simulink model "projet_RST_lineaire"  (R2023a)
settings: Solver=VariableStepAuto  StartTime=0.0  StopTime=1  RelTol=1e-3
undefined symbols (not defined in the file): R, S, T, Te
libraries: cstblocks x2
settings Model: Creator=leolebuhotel  LastModifiedBy=leolebuhotel

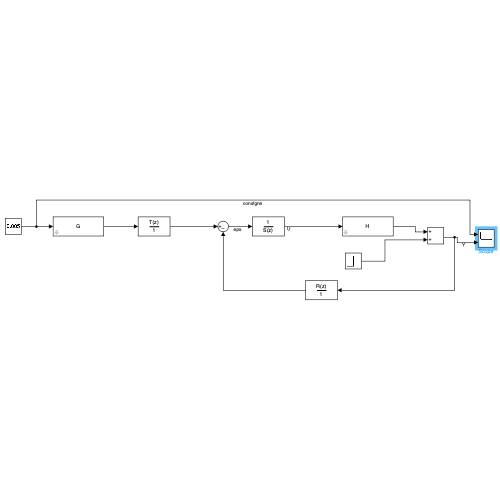
[thumbnail: Simulink's stored preview of the top-level diagram]
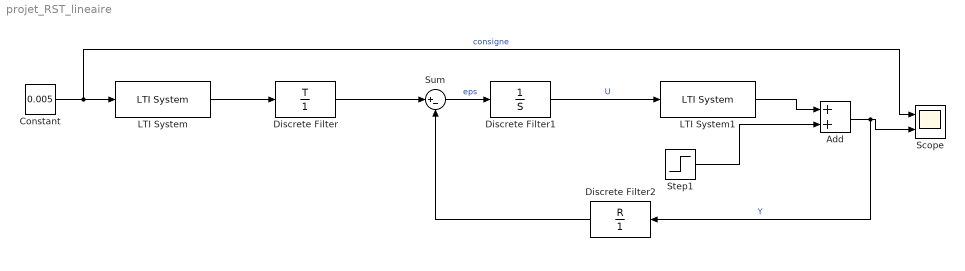
== system projet_RST_lineaire ==
  Add : Sum
  Constant : Constant  Value=0.005
  Discrete Filter : DiscreteFilter  Numerator=T  Denominator=1  SampleTime=Te
  Discrete Filter1 : DiscreteFilter  Numerator=1  Denominator=S  SampleTime=Te
  Discrete Filter2 : DiscreteFilter  Numerator=R  Denominator=1
  LTI System : cstblocks/LTI System  sys=G  IC=[]
  LTI System1 : cstblocks/LTI System  sys=H  IC=[]
  Scope : Scope  NumInputPorts=2
  Step1 : Step  Time=0.5  After=0.002  SampleTime=0
  Sum : Sum  Inputs=|+-
  wires:
  Discrete Filter2/1 -> Sum/2
  Sum/1 -> Discrete Filter1/1  "eps"
  Discrete Filter/1 -> Sum/1
  LTI System/1 -> Discrete Filter/1
  Constant/1 -> Scope/1, LTI System/1  "consigne"
  Step1/1 -> Add/2
  Add/1 -> Discrete Filter2/1, Scope/2  "Y"
  Discrete Filter1/1 -> LTI System1/1  "U"
  LTI System1/1 -> Add/1
